simulink model "rocket_3dof_realistic"  (R2026a)
settings: Solver=VariableStepAuto  StopTime=60
undefined symbols (not defined in the file): g, Iyy, Kvx, Kvz, Kx, Kz, lever_arm, m
libraries: slpidlib x1
settings Model: Creator=shane.zins  LastModifiedBy=shane.zins

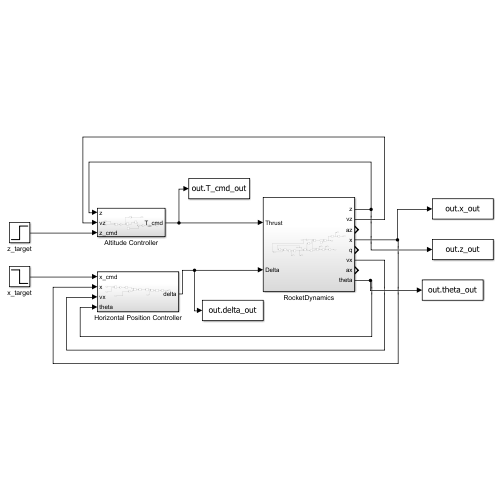
[thumbnail: Simulink's stored preview of the top-level diagram]
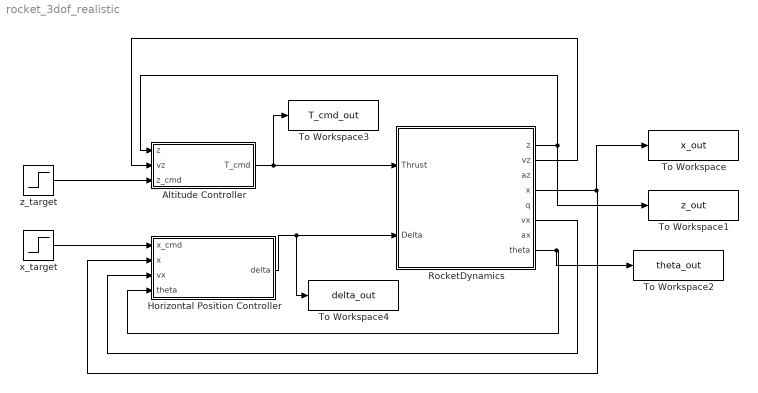
== system rocket_3dof_realistic ==
  Altitude Controller : Subsystem
  Horizontal Position Controller : Subsystem
  RocketDynamics : Subsystem
  To Workspace : ToWorkspace  VariableName=x_out  SaveFormat=Timeseries  SampleTime=-1
  To Workspace1 : ToWorkspace  VariableName=z_out  SaveFormat=Timeseries  SampleTime=-1
  To Workspace2 : ToWorkspace  VariableName=theta_out  SaveFormat=Timeseries  SampleTime=-1
  To Workspace3 : ToWorkspace  VariableName=T_cmd_out  SaveFormat=Timeseries  SampleTime=-1
  To Workspace4 : ToWorkspace  VariableName=delta_out  SaveFormat=Timeseries  SampleTime=-1
  x_target : Step  FinalValue=x_target  SampleTime=0
  z_target : Step  FinalValue=z_target  SampleTime=0
  wires:
  RocketDynamics/1(z) -> To Workspace1/1, Altitude Controller/1(z)
  RocketDynamics/4(x) -> To Workspace/1, Horizontal Position Controller/2(x)
  RocketDynamics/2(vz) -> Altitude Controller/2(vz)
  z_target/1 -> Altitude Controller/3(z_cmd)
  Altitude Controller/1(T_cmd) -> To Workspace3/1, RocketDynamics/1(Thrust)
  Horizontal Position Controller/1(delta) -> To Workspace4/1, RocketDynamics/2(Delta)
  x_target/1 -> Horizontal Position Controller/1(x_cmd)
  RocketDynamics/6(vx) -> Horizontal Position Controller/3(vx)
  RocketDynamics/8(theta) -> To Workspace2/1, Horizontal Position Controller/4(theta)

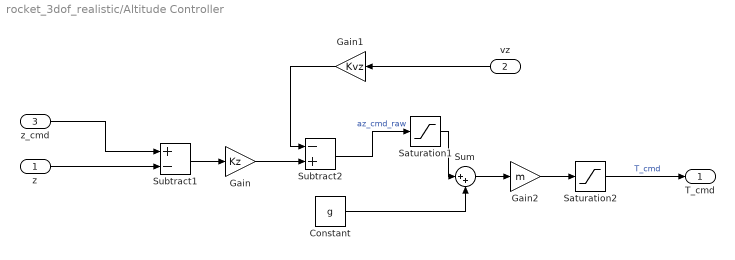
== system rocket_3dof_realistic/Altitude Controller ==
  z : Inport
  vz : Inport  Port=2
  z_cmd : Inport  Port=3
  Constant : Constant  Value=g
  Gain : Gain  Gain=Kz
  Gain1 : Gain  Gain=Kvz
  Gain2 : Gain  Gain=m
  Saturation1 : Saturate  UpperLimit=5  LowerLimit=-5
  Saturation2 : Saturate  UpperLimit=2000  LowerLimit=0
  Subtract1 : Sum  Inputs=+-
  Subtract2 : Sum  Inputs=-+
  Sum : Sum  Inputs=|++
  T_cmd : Outport
  wires:
  Gain2/1 -> Saturation2/1
  Saturation1/1 -> Sum/1
  vz/1 -> Gain1/1
  Subtract1/1 -> Gain/1
  Gain/1 -> Subtract2/2
  Saturation2/1 -> T_cmd/1  "T_cmd"
  Gain1/1 -> Subtract2/1
  Sum/1 -> Gain2/1
  Subtract2/1 -> Saturation1/1  "az_cmd_raw"
  Constant/1 -> Sum/2
  z/1 -> Subtract1/2
  z_cmd/1 -> Subtract1/1

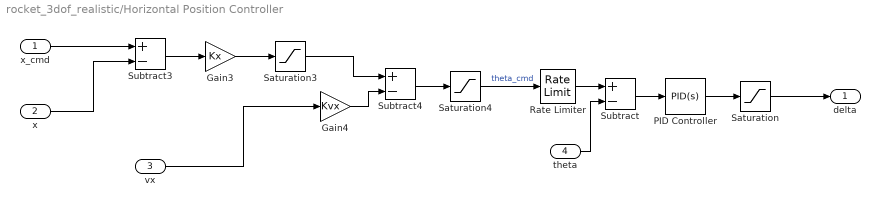
== system rocket_3dof_realistic/Horizontal Position Controller ==
  x_cmd : Inport
  x : Inport  Port=2
  vx : Inport  Port=3
  theta : Inport  Port=4
  Gain3 : Gain  Gain=Kx
  Gain4 : Gain  Gain=Kvx
  PID Controller : slpidlib/PID Controller  Controller=PID  Form=Parallel  TimeDomain=Continuous-time  UseExternalTs=off  SampleTime=-1  IntegratorMethod=Forward Euler  FilterMethod=Forward Euler  ControllerParametersSource=internal  P=0.096975521172559  I=0  UseKiTs=off  D=0.35  UseExternalDerivativeSource=off  N=261.806764299177  UseFilter=on  TunerSelectOption=Transfer Function Based (PID Tuner App)  InitialConditionSource=internal  InitialConditionForIntegrator=0  InitialConditionForFilter=0  DifferentiatorICPrevScaledInput=0  ExternalReset=none  TrackingMode=off  Kt=1  LimitOutput=off  SatLimitsSource=internal  UpperSaturationLimit=0.2  LowerSaturationLimit=-0.2  LinearizeAsGain=on  AntiWindupMode=back-calculation  Kb=1  LimitIntegrator=off  UpperIntegratorSaturationLimit=inf  LowerIntegratorSaturationLimit=-inf  POutMin=[]  POutMax=[]  IOutMin=[]  IOutMax=[]  DOutMin=[]  DOutMax=[]  NOutMin=[]  NOutMax=[]  SumOutMin=[]  SumOutMax=[]  SaturationOutMin=[]  SaturationOutMax=[]  PParamMin=[]  PParamMax=[]  IParamMin=[]  IParamMax=[]  DParamMin=[]  DParamMax=[]  NParamMin=[]  NParamMax=[]  KbParamMin=[]  KbParamMax=[]  KtParamMin=[]  KtParamMax=[]  KbOutMin=[]  KbOutMax=[]  KtOutMin=[]  KtOutMax=[]  IntegratorOutMin=[]  IntegratorOutMax=[]  FilterOutMin=[]  FilterOutMax=[]  SumI1OutMin=[]  SumI1OutMax=[]  SumI2OutMin=[]  SumI2OutMax=[]  SumI3OutMin=[]  SumI3OutMax=[]  SumI4OutMin=[]  SumI4OutMax=[]  SumDOutMin=[]  SumDOutMax=[]  DifferentiatorOutMin=[]  DifferentiatorOutMax=[]  FilterDiffOutCoefMin=[]  FilterDiffOutCoefMax=[]  ReciprocalOutMin=[]  ReciprocalOutMax=[]  SumDenOutMin=[]  SumDenOutMax=[]  SumNumOutMin=[]  SumNumOutMax=[]  DivideOutMin=[]  DivideOutMax=[]  UdiffTsProdOutMin=[]  UdiffTsProdOutMax=[]  NTsProdOutMin=[]  NTsProdOutMax=[]  UintegralTsProdOutMin=[]  UintegralTsProdOutMax=[]  UngainTsProdOutMin=[]  UngainTsProdOutMax=[]  ClampingZeroOutDataTypeStr=Inherit: Inherit via back propagation  ClampingZeroOutMin=[]  ClampingZeroOutMax=[]  FilterDenConstantOutDataTypeStr=Inherit: Inherit via back propagation  FilterDenConstantOutMin=[]  FilterDenConstantOutMax=[]  PCopyOutDataTypeStr=Inherit: Inherit via back propagation  PCopyOutMin=[]  PCopyOutMax=[]  NCopyOutDataTypeStr=Inherit: Inherit via back propagation  NCopyOutMin=[]  NCopyOutMax=[]  IntegratorContinuousStateAttributes=''  IntegratorStateMustResolveToSignalObject=off  IntegratorRTWStateStorageClass=Auto  FilterContinuousStateAttributes=''  FilterStateMustResolveToSignalObject=off  FilterRTWStateStorageClass=Auto  ParallelPVariant=InternalParameters  IdealPVariant=Disabled  IVariant=InternalParameters  DVariant=InternalParameters  IntegratorVariant=Continuous  SatVariant=Disabled  AWVariant=Passthrough  PCopyVariant=Disabled  TRVariant=Disabled  FdbkBlocksVariant=Forward  IdealPFdbkVariant=Disabled  SatFdbkVariant=Disabled  DerivativeFilterVariant=ContFilter  NVariant=InternalParameters  NCopyVariant=Disabled  FilterICVariant=InternalICsFilter  IntegratorICVariant=InternalICs  ExternalResetVariant=Disabled  TRSumVariant=Passthrough  SumFdbkVariant=Disabled  SumVariant=Sum_PID  TsampFilterVariant=InternalTs  TsampNgainVariant=Passthrough  TsampIntegralVariant=Disabled_SignalSpec  ExternalSaturationOutDataTypeStr=Inherit: Same as second input  DerivativeSourceVariant=ErrorSignal  PreIntVariant=InternalPreInt
  Rate Limiter : RateLimiter  RisingSlewLimit=0.05  FallingSlewLimit=-0.05  SampleTimeMode=inherited
  Saturation : Saturate  UpperLimit=0.2  LowerLimit=-0.2
  Saturation3 : Saturate  UpperLimit=0.1745  LowerLimit=-0.1745
  Saturation4 : Saturate  UpperLimit=deg2rad(10)  LowerLimit=-deg2rad(10)
  Subtract : Sum  Inputs=+-
  Subtract3 : Sum  Inputs=+-
  Subtract4 : Sum  Inputs=+-
  delta : Outport
  wires:
  Gain4/1 -> Subtract4/2
  Saturation3/1 -> Subtract4/1
  Saturation4/1 -> Rate Limiter/1  "theta_cmd"
  Subtract4/1 -> Saturation4/1
  Gain3/1 -> Saturation3/1
  x_cmd/1 -> Subtract3/1
  Subtract3/1 -> Gain3/1
  Rate Limiter/1 -> Subtract/1
  PID Controller/1 -> Saturation/1
  Subtract/1 -> PID Controller/1
  x/1 -> Subtract3/2
  vx/1 -> Gain4/1
  Saturation/1 -> delta/1
  theta/1 -> Subtract/2

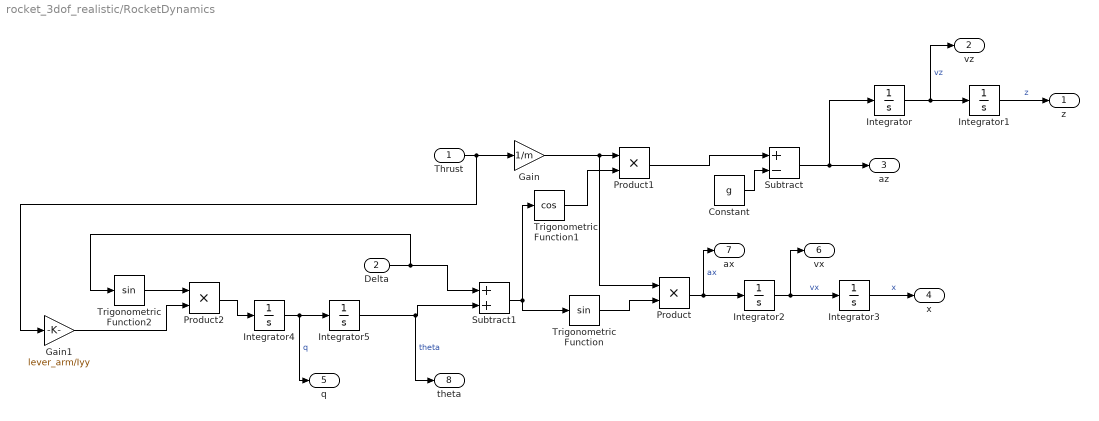
== system rocket_3dof_realistic/RocketDynamics ==
  Thrust : Inport
  Delta : Inport  Port=2
  Constant : Constant  Value=g
  Gain : Gain  Gain=1/m
  Gain1 : Gain  Gain=lever_arm/Iyy
  Integrator{,1..5} (6 alike) : Integrator
  Product : Product
  Product1 : Product
  Product2 : Product
  Subtract : Sum  Inputs=+-
  Subtract1 : Sum
  Trigonometric Function : Trigonometry
  Trigonometric Function1 : Trigonometry  Operator=cos
  Trigonometric Function2 : Trigonometry
  z : Outport
  vz : Outport  Port=2
  az : Outport  Port=3
  x : Outport  Port=4
  q : Outport  Port=5
  vx : Outport  Port=6
  ax : Outport  Port=7
  theta : Outport  Port=8
  wires:
  Integrator/1 -> Integrator1/1, vz/1  "vz"
  Integrator1/1 -> z/1  "z"
  Thrust/1 -> Gain1/1, Gain/1
  Subtract/1 -> Integrator/1, az/1
  Integrator2/1 -> vx/1, Integrator3/1  "vx"
  Integrator3/1 -> x/1  "x"
  Trigonometric Function/1 -> Product/2
  Constant/1 -> Subtract/2
  Product/1 -> ax/1, Integrator2/1  "ax"
  Delta/1 -> Trigonometric Function2/1, Subtract1/1
  Subtract1/1 -> Trigonometric Function/1, Trigonometric Function1/1
  Gain/1 -> Product1/1, Product/1
  Trigonometric Function1/1 -> Product1/2
  Product1/1 -> Subtract/1
  Integrator4/1 -> q/1, Integrator5/1  "q"
  Integrator5/1 -> theta/1, Subtract1/2  "theta"
  Trigonometric Function2/1 -> Product2/1
  Gain1/1 -> Product2/2
  Product2/1 -> Integrator4/1
